simulink model "ActuatorRatingModel"  (R2024a)
settings: Solver=VariableStepAuto  StartTime=0.0  StopTime=simT  MaxStep=1e-3  MinStep=1e-4  RelTol=1e-3
PostLoadFcn:
  | run('ParametricRobotParameters')
  | run('ParametricGripperPayloadsParameters.m');
  | simT = 2;
  | load('configModelWorkspace.mat');
  | jointDataBus = jointDataBusCreator;
undefined symbols (not defined in the file): ParametricRobot, positionLimits, timeScale, velocityLimits, waypoints, X, Y, Z
libraries: nesl_utility x7, simulink x6, sm_lib x4
settings Model: Creator=jjha  LastModifiedBy=abirdas
settings OptimizationCC: ReuseModelBlockBuffer=off
settings RTWCC: GPUComputeCapability=3.5
settings SimscapeCC: SimscapeLogType=all

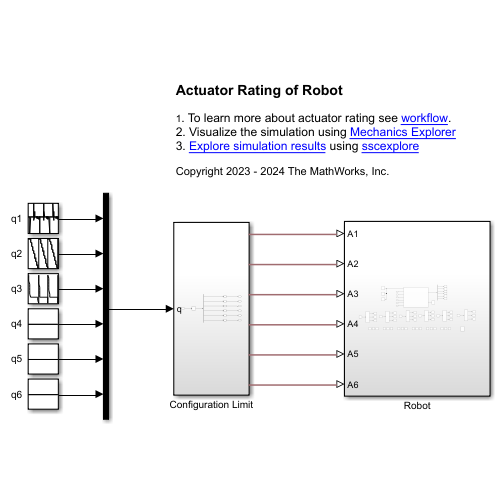
[thumbnail: Simulink's stored preview of the top-level diagram]
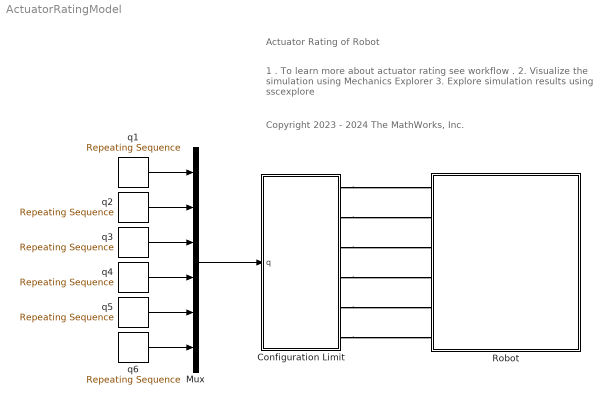
== system ActuatorRatingModel ==
  note: Copyright 2023 - 2024 The MathWorks, Inc.
  note: Actuator Rating of Robot
  note: 1 . To learn more about actuator rating see workflow .
      | 2. Visualize the simulation using Mechanics Explorer
      | 3. Explore simulation results using sscexplore
  Configuration Limit : Subsystem
  Mux : Mux  Inputs=6
  Robot : Subsystem
  q1 : simulink/Sources/Repeating Sequence  rep_seq_t=[1 : length(waypoints)] * timeScale  rep_seq_y=waypoints(1,:)
  q2 : simulink/Sources/Repeating Sequence  rep_seq_t=[1 : length(waypoints)] * timeScale  rep_seq_y=waypoints(2,:)
  q3 : simulink/Sources/Repeating Sequence  rep_seq_t=[1 : length(waypoints)] * timeScale  rep_seq_y=waypoints(3,:)
  q4 : simulink/Sources/Repeating Sequence  rep_seq_t=[1 : length(waypoints)] * timeScale  rep_seq_y=waypoints(4,:)
  q5 : simulink/Sources/Repeating Sequence  rep_seq_t=[1 : length(waypoints)] * timeScale  rep_seq_y=waypoints(5,:)
  q6 : simulink/Sources/Repeating Sequence  rep_seq_t=[1 : length(waypoints)] * timeScale  rep_seq_y=waypoints(6,:)
  wires:
  q1/1 -> Mux/1
  Mux/1 -> Configuration Limit/1(q)
  q6/1 -> Mux/6
  q3/1 -> Mux/3
  q5/1 -> Mux/5
  q2/1 -> Mux/2
  q4/1 -> Mux/4
  connections:
  Configuration Limit/RConn5 -- Robot/LConn5
  Configuration Limit/RConn6 -- Robot/LConn6
  Configuration Limit/RConn4 -- Robot/LConn4
  Configuration Limit/RConn1 -- Robot/LConn1
  Configuration Limit/RConn3 -- Robot/LConn3
  Configuration Limit/RConn2 -- Robot/LConn2

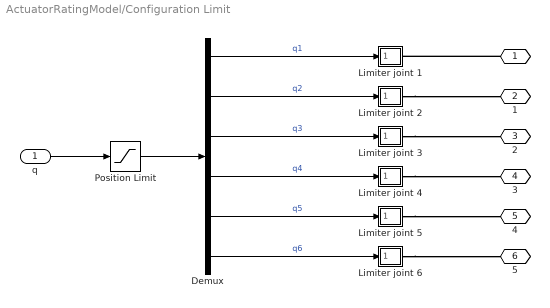
== system ActuatorRatingModel/Configuration Limit ==
  q : Inport
  Demux : Demux  Outputs=6
  Limiter joint 1 : Subsystem  mask(Limiter){maxVel=velocityLimits(1), maxAcc=0.1}
      mask prompts: maxVel "Max velocity of joint (rad/s)"; maxAcc "max acceleration of joint (rad/s^2)"
      mask help: Limit the velocity and acceleration of joints.
      mask DialogControl ParameterGroupVar Prompt: Limits
  Limiter joint 2 : Subsystem  mask(Limiter){maxVel=velocityLimits(2), maxAcc=0.1}
      mask prompts: maxVel "Max velocity of joint (rad/s)"; maxAcc "max acceleration of joint (rad/s^2)"
      mask help: Limit the velocity and acceleration of joints.
      mask DialogControl ParameterGroupVar Prompt: Limits
  Limiter joint 3 : Subsystem  mask(Limiter){maxVel=velocityLimits(3), maxAcc=0.1}
      mask prompts: maxVel "Max velocity of joint (rad/s)"; maxAcc "max acceleration of joint (rad/s^2)"
      mask help: Limit the velocity and acceleration of joints.
      mask DialogControl ParameterGroupVar Prompt: Limits
  Limiter joint 4 : Subsystem  mask(Limiter){maxVel=velocityLimits(4), maxAcc=0.1}
      mask prompts: maxVel "Max velocity of joint (rad/s)"; maxAcc "max acceleration of joint (rad/s^2)"
      mask help: Limit the velocity and acceleration of joints.
      mask DialogControl ParameterGroupVar Prompt: Limits
  Limiter joint 5 : Subsystem  mask(Limiter){maxVel=velocityLimits(5), maxAcc=0.1}
      mask prompts: maxVel "Max velocity of joint (rad/s)"; maxAcc "max acceleration of joint (rad/s^2)"
      mask help: Limit the velocity and acceleration of joints.
      mask DialogControl ParameterGroupVar Prompt: Limits
  Limiter joint 6 : Subsystem  mask(Limiter){maxVel=velocityLimits(6), maxAcc=0.1}
      mask prompts: maxVel "Max velocity of joint (rad/s)"; maxAcc "max acceleration of joint (rad/s^2)"
      mask help: Limit the velocity and acceleration of joints.
      mask DialogControl ParameterGroupVar Prompt: Limits
  Position Limit : Saturate  UpperLimit=positionLimits(:, 2)  LowerLimit=positionLimits(:, 1)
  " " : PMIOPort  Side=Right
  " 1" : PMIOPort  Port=2  Side=Right
  " 2" : PMIOPort  Port=3  Side=Right
  " 3" : PMIOPort  Port=4  Side=Right
  " 4" : PMIOPort  Port=5  Side=Right
  " 5" : PMIOPort  Port=6  Side=Right
  wires:
  Demux/1 -> Limiter joint 1/1(" ")  "q1"
  q/1 -> Position Limit/1
  Demux/2 -> Limiter joint 2/1(" ")  "q2"
  Demux/3 -> Limiter joint 3/1(" ")  "q3"
  Demux/4 -> Limiter joint 4/1(" ")  "q4"
  Demux/5 -> Limiter joint 5/1(" ")  "q5"
  Demux/6 -> Limiter joint 6/1(" ")  "q6"
  Position Limit/1 -> Demux/1
  connections:
  " "/RConn1 -- Limiter joint 1/RConn1
  Limiter joint 2/RConn1 -- " 1"/RConn1
  Limiter joint 3/RConn1 -- " 2"/RConn1
  Limiter joint 4/RConn1 -- " 3"/RConn1
  Limiter joint 5/RConn1 -- " 4"/RConn1
  Limiter joint 6/RConn1 -- " 5"/RConn1

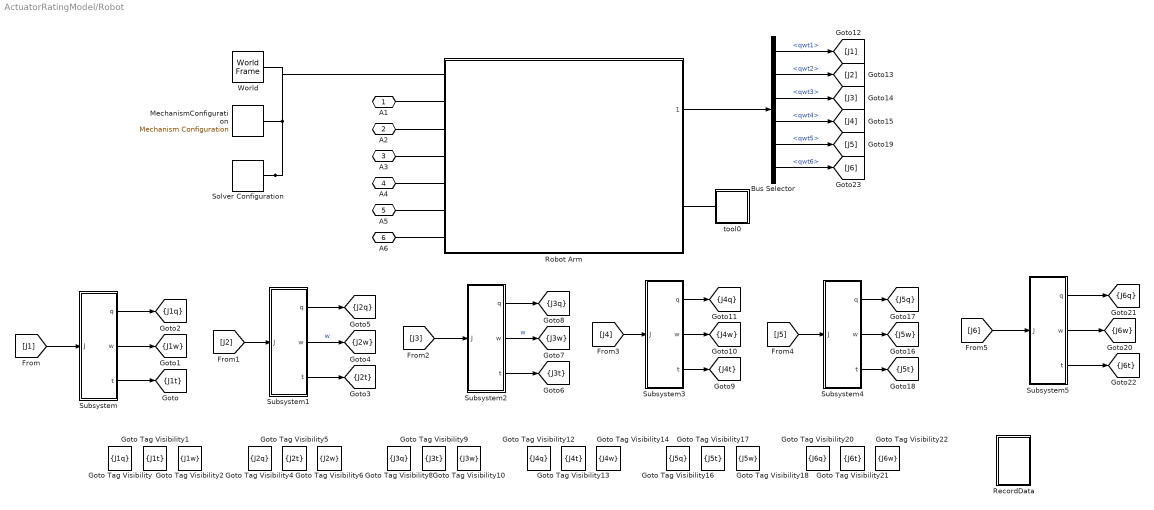
== system ActuatorRatingModel/Robot ==
  Bus Selector : BusSelector  OutputSignals=qwt1,qwt2,qwt3,qwt4,qwt5,qwt6
  Goto Tag Visibility : GotoTagVisibility  GotoTag=J1q
  Goto Tag Visibility1 : GotoTagVisibility  GotoTag=J1t
  Goto Tag Visibility10 : GotoTagVisibility  GotoTag=J3w
  Goto Tag Visibility12 : GotoTagVisibility  GotoTag=J4q
  Goto Tag Visibility13 : GotoTagVisibility  GotoTag=J4t
  Goto Tag Visibility14 : GotoTagVisibility  GotoTag=J4w
  Goto Tag Visibility16 : GotoTagVisibility  GotoTag=J5q
  Goto Tag Visibility17 : GotoTagVisibility  GotoTag=J5t
  Goto Tag Visibility18 : GotoTagVisibility  GotoTag=J5w
  Goto Tag Visibility2 : GotoTagVisibility  GotoTag=J1w
  Goto Tag Visibility20 : GotoTagVisibility  GotoTag=J6q
  Goto Tag Visibility21 : GotoTagVisibility  GotoTag=J6t
  Goto Tag Visibility22 : GotoTagVisibility  GotoTag=J6w
  Goto Tag Visibility4 : GotoTagVisibility  GotoTag=J2q
  Goto Tag Visibility5 : GotoTagVisibility  GotoTag=J2t
  Goto Tag Visibility6 : GotoTagVisibility  GotoTag=J2w
  Goto Tag Visibility8 : GotoTagVisibility  GotoTag=J3q
  Goto Tag Visibility9 : GotoTagVisibility  GotoTag=J3t
  MechanismConfiguration : sm_lib/Utilities/Mechanism Configuration  UniformGravity=Constant  GravityVector=[0 0 -9.80665]  GravityVectorUnits=m/s^2  LinearizationDelta=0.001  JointModeTransitionNonlinearIterations=2
  RecordData : Subsystem
  Robot Arm : Subsystem  ReferencedSubsystem=ParametricRobotSubsystem  workflow=ones(1,6)*2
  Solver Configuration : nesl_utility/Solver Configuration  PhysicalDomain=network_engine_domain  SubClassName=solver  LeftPortType=input  RightPortType=generic  Tones=[]  Harmonics=[]  SimulateNoise=off  Profile=off  UseLocalSampling=off  EnableSwitchedLinearOptims=on  FrequencyDomain=off  UseCCode=off  RelTol=0.001  AbsTol=0.001  MinStep=1e-09  ToWorkspace=off  RevertToSquareIcSolve=off  NumHomotopyIterations=100  PhasorMode=off  PhasorModeNumHarmonics=1  ConsistencySolver=NEWTON_XTOL_AFTER_FTOL  IndexReductionMethod=DerivativeReplacement  DoDC=off  ResidualTolerance=1e-09  ConsistencyTolSource=GLOBAL  ConsistencyAbsTol=0.001  ConsistencyRelTol=0.001  ConsistencyTolFactor=0.001  UseLocalSolver=off  LocalSolverChoice=NE_BACKWARD_EULER_ADVANCER  ResolveIndetEquations=on  FunctionEvalNumThread=1  LocalSolverSampleTime=0.001  DoFixedCost=off  MaxNonlinIter=3  MaxModeIter=2  ComputeImpulses=off  ImpulseIterations=2  LinearAlgebra=auto  LinearAlgebraNumThread=0  EquationFormulation=NE_TIME_EF  DelaysMemoryBudget=1024  AutomaticFiltering=on  FilteringTimeConstant=0.001  PartitionStorageMethod=AS_NEEDED  PartitionMemoryBudget=1024  PartitionMethod=ROBUST  MultibodyUseLocalSolver=off  MultibodyLocalSolverChoice=ODE1  MultibodyLocalSolverSampleTime=0.001
  Subsystem : Subsystem
  Subsystem1 : Subsystem
  Subsystem2 : Subsystem
  Subsystem3 : Subsystem
  Subsystem4 : Subsystem
  Subsystem5 : Subsystem
  World : sm_lib/Frames and Transforms/World Frame
  tool0 : Subsystem
  A1 : PMIOPort  Side=Left
  A2 : PMIOPort  Port=2  Side=Left
  A3 : PMIOPort  Port=3  Side=Left
  A4 : PMIOPort  Port=4  Side=Left
  A5 : PMIOPort  Port=5  Side=Left
  A6 : PMIOPort  Port=6  Side=Left
  tag scope: J1q=scoped, J1t=scoped, J1w=scoped, J2q=scoped, J2t=scoped, J2w=scoped, J3q=scoped, J3t=scoped, J3w=scoped, J4q=scoped, J4t=scoped, J4w=scoped, J5q=scoped, J5t=scoped, J5w=scoped, J6q=scoped, J6t=scoped, J6w=scoped
  wires:
  Subsystem4/1(q) -> [J5q]
  Subsystem/2(w) -> [J1w]
  Subsystem5/2(w) -> [J6w]
  [J4] -> Subsystem3/1(J)
  Subsystem5/3(t) -> [J6t]
  Subsystem/3(t) -> [J1t]
  Subsystem4/2(w) -> [J5w]
  [J6] -> Subsystem5/1(J)
  [J3] -> Subsystem2/1(J)
  Subsystem5/1(q) -> [J6q]
  Subsystem1/1(q) -> [J2q]
  [J1] -> Subsystem/1(J)
  [J2] -> Subsystem1/1(J)
  Subsystem/1(q) -> [J1q]
  Subsystem3/1(q) -> [J4q]
  Subsystem3/2(w) -> [J4w]
  Subsystem4/3(t) -> [J5t]
  Subsystem2/1(q) -> [J3q]
  Subsystem2/2(w) -> [J3w]  "w"
  [J5] -> Subsystem4/1(J)
  Subsystem2/3(t) -> [J3t]
  Subsystem1/2(w) -> [J2w]  "w"
  Subsystem1/3(t) -> [J2t]
  Subsystem3/3(t) -> [J4t]
  Bus Selector/1 -> [J1]  "<qwt1>"
  Bus Selector/2 -> [J2]  "<qwt2>"
  Bus Selector/3 -> [J3]  "<qwt3>"
  Bus Selector/4 -> [J4]  "<qwt4>"
  Bus Selector/5 -> [J5]  "<qwt5>"
  Bus Selector/6 -> [J6]  "<qwt6>"
  Robot Arm/1 -> Bus Selector/1
  connections:
  Solver Configuration/RConn1 -- Robot Arm/LConn1 -- World/RConn1 -- MechanismConfiguration/RConn1
  A5/RConn1 -- Robot Arm/LConn6
  tool0/LConn1 -- Robot Arm/RConn1
  A4/RConn1 -- Robot Arm/LConn5
  A3/RConn1 -- Robot Arm/LConn4
  A1/RConn1 -- Robot Arm/LConn2
  A2/RConn1 -- Robot Arm/LConn3
  A6/RConn1 -- Robot Arm/LConn7

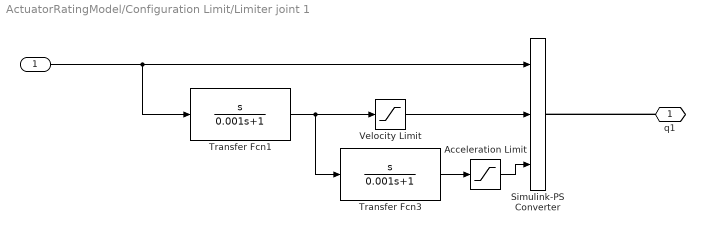
== system ActuatorRatingModel/Configuration Limit/Limiter joint 1 ==
  " " : Inport
  Acceleration Limit : Saturate  UpperLimit=maxAcc  LowerLimit=-maxAcc
  Simulink-PS Converter : nesl_utility/Simulink-PS Converter  PhysicalDomain=network_engine_domain  SubClassName=ps_input  LeftPortType=input  RightPortType=output  PseudoPeriodic=off  Frequencies=[]  NoiseDistribution=none  NoiseParameters=[]  Unit=rad  AffineConversion=off  FilteringAndDerivatives=provide  SimscapeFilterOrder=1  InputFilterTimeConstant=0.001  UdotUserProvided=2
  Transfer Fcn1 : TransferFcn  Numerator=[1 0]  Denominator=[0.001 1]
  Transfer Fcn3 : TransferFcn  Numerator=[1 0]  Denominator=[0.001 1]
  Velocity Limit : Saturate  UpperLimit=maxVel  LowerLimit=-maxVel
  q1 : PMIOPort  Side=Right
  wires:
  " "/1 -> Transfer Fcn1/1, Simulink-PS Converter/1
  Transfer Fcn1/1 -> Transfer Fcn3/1, Velocity Limit/1
  Velocity Limit/1 -> Simulink-PS Converter/2
  Transfer Fcn3/1 -> Acceleration Limit/1
  Acceleration Limit/1 -> Simulink-PS Converter/3
  connections:
  q1/RConn1 -- Simulink-PS Converter/RConn1

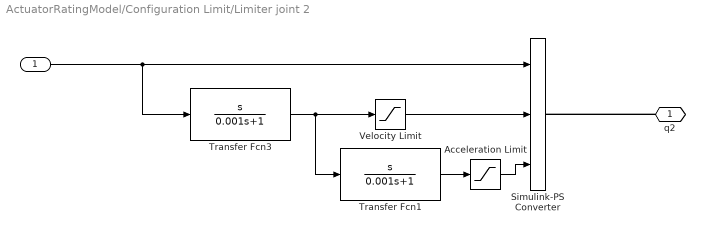
== system ActuatorRatingModel/Configuration Limit/Limiter joint 2 ==
  " " : Inport
  Acceleration Limit : Saturate  UpperLimit=maxAcc  LowerLimit=-maxAcc
  Simulink-PS Converter : nesl_utility/Simulink-PS Converter  PhysicalDomain=network_engine_domain  SubClassName=ps_input  LeftPortType=input  RightPortType=output  PseudoPeriodic=off  Frequencies=[]  NoiseDistribution=none  NoiseParameters=[]  Unit=rad  AffineConversion=off  FilteringAndDerivatives=provide  SimscapeFilterOrder=1  InputFilterTimeConstant=0.001  UdotUserProvided=2
  Transfer Fcn1 : TransferFcn  Numerator=[1 0]  Denominator=[0.001 1]
  Transfer Fcn3 : TransferFcn  Numerator=[1 0]  Denominator=[0.001 1]
  Velocity Limit : Saturate  UpperLimit=maxVel  LowerLimit=-maxVel
  q2 : PMIOPort  Side=Right
  wires:
  Transfer Fcn1/1 -> Acceleration Limit/1
  Transfer Fcn3/1 -> Transfer Fcn1/1, Velocity Limit/1
  " "/1 -> Transfer Fcn3/1, Simulink-PS Converter/1
  Velocity Limit/1 -> Simulink-PS Converter/2
  Acceleration Limit/1 -> Simulink-PS Converter/3
  connections:
  q2/RConn1 -- Simulink-PS Converter/RConn1

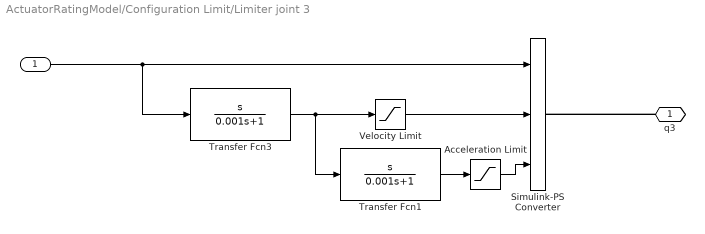
== system ActuatorRatingModel/Configuration Limit/Limiter joint 3 ==
  " " : Inport
  Acceleration Limit : Saturate  UpperLimit=maxAcc  LowerLimit=-maxAcc
  Simulink-PS Converter : nesl_utility/Simulink-PS Converter  PhysicalDomain=network_engine_domain  SubClassName=ps_input  LeftPortType=input  RightPortType=output  PseudoPeriodic=off  Frequencies=[]  NoiseDistribution=none  NoiseParameters=[]  Unit=rad  AffineConversion=off  FilteringAndDerivatives=provide  SimscapeFilterOrder=1  InputFilterTimeConstant=0.001  UdotUserProvided=2
  Transfer Fcn1 : TransferFcn  Numerator=[1 0]  Denominator=[0.001 1]
  Transfer Fcn3 : TransferFcn  Numerator=[1 0]  Denominator=[0.001 1]
  Velocity Limit : Saturate  UpperLimit=maxVel  LowerLimit=-maxVel
  q3 : PMIOPort  Side=Right
  wires:
  " "/1 -> Transfer Fcn3/1, Simulink-PS Converter/1
  Transfer Fcn3/1 -> Transfer Fcn1/1, Velocity Limit/1
  Velocity Limit/1 -> Simulink-PS Converter/2
  Transfer Fcn1/1 -> Acceleration Limit/1
  Acceleration Limit/1 -> Simulink-PS Converter/3
  connections:
  q3/RConn1 -- Simulink-PS Converter/RConn1

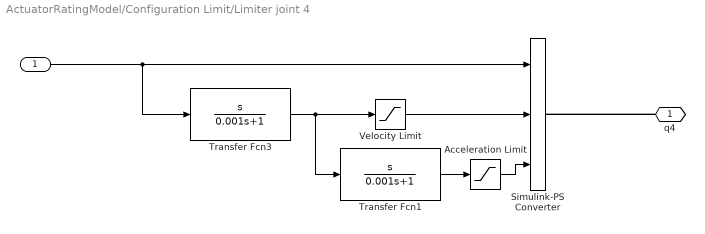
== system ActuatorRatingModel/Configuration Limit/Limiter joint 4 ==
  " " : Inport
  Acceleration Limit : Saturate  UpperLimit=maxAcc  LowerLimit=-maxAcc
  Simulink-PS Converter : nesl_utility/Simulink-PS Converter  PhysicalDomain=network_engine_domain  SubClassName=ps_input  LeftPortType=input  RightPortType=output  PseudoPeriodic=off  Frequencies=[]  NoiseDistribution=none  NoiseParameters=[]  Unit=rad  AffineConversion=off  FilteringAndDerivatives=provide  SimscapeFilterOrder=1  InputFilterTimeConstant=0.001  UdotUserProvided=2
  Transfer Fcn1 : TransferFcn  Numerator=[1 0]  Denominator=[0.001 1]
  Transfer Fcn3 : TransferFcn  Numerator=[1 0]  Denominator=[0.001 1]
  Velocity Limit : Saturate  UpperLimit=maxVel  LowerLimit=-maxVel
  q4 : PMIOPort  Side=Right
  wires:
  Acceleration Limit/1 -> Simulink-PS Converter/3
  Transfer Fcn1/1 -> Acceleration Limit/1
  Velocity Limit/1 -> Simulink-PS Converter/2
  Transfer Fcn3/1 -> Transfer Fcn1/1, Velocity Limit/1
  " "/1 -> Transfer Fcn3/1, Simulink-PS Converter/1
  connections:
  q4/RConn1 -- Simulink-PS Converter/RConn1

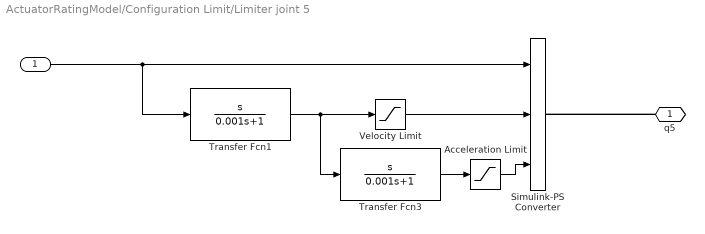
== system ActuatorRatingModel/Configuration Limit/Limiter joint 5 ==
  " " : Inport
  Acceleration Limit : Saturate  UpperLimit=maxAcc  LowerLimit=-maxAcc
  Simulink-PS Converter : nesl_utility/Simulink-PS Converter  PhysicalDomain=network_engine_domain  SubClassName=ps_input  LeftPortType=input  RightPortType=output  PseudoPeriodic=off  Frequencies=[]  NoiseDistribution=none  NoiseParameters=[]  Unit=rad  AffineConversion=off  FilteringAndDerivatives=provide  SimscapeFilterOrder=1  InputFilterTimeConstant=0.001  UdotUserProvided=2
  Transfer Fcn1 : TransferFcn  Numerator=[1 0]  Denominator=[0.001 1]
  Transfer Fcn3 : TransferFcn  Numerator=[1 0]  Denominator=[0.001 1]
  Velocity Limit : Saturate  UpperLimit=maxVel  LowerLimit=-maxVel
  q5 : PMIOPort  Side=Right
  wires:
  " "/1 -> Transfer Fcn1/1, Simulink-PS Converter/1
  Transfer Fcn1/1 -> Transfer Fcn3/1, Velocity Limit/1
  Velocity Limit/1 -> Simulink-PS Converter/2
  Transfer Fcn3/1 -> Acceleration Limit/1
  Acceleration Limit/1 -> Simulink-PS Converter/3
  connections:
  q5/RConn1 -- Simulink-PS Converter/RConn1

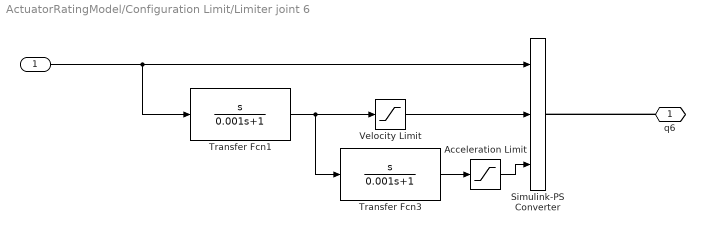
== system ActuatorRatingModel/Configuration Limit/Limiter joint 6 ==
  " " : Inport
  Acceleration Limit : Saturate  UpperLimit=maxAcc  LowerLimit=-maxAcc
  Simulink-PS Converter : nesl_utility/Simulink-PS Converter  PhysicalDomain=network_engine_domain  SubClassName=ps_input  LeftPortType=input  RightPortType=output  PseudoPeriodic=off  Frequencies=[]  NoiseDistribution=none  NoiseParameters=[]  Unit=rad  AffineConversion=off  FilteringAndDerivatives=provide  SimscapeFilterOrder=1  InputFilterTimeConstant=0.001  UdotUserProvided=2
  Transfer Fcn1 : TransferFcn  Numerator=[1 0]  Denominator=[0.001 1]
  Transfer Fcn3 : TransferFcn  Numerator=[1 0]  Denominator=[0.001 1]
  Velocity Limit : Saturate  UpperLimit=maxVel  LowerLimit=-maxVel
  q6 : PMIOPort  Side=Right
  wires:
  Acceleration Limit/1 -> Simulink-PS Converter/3
  Transfer Fcn3/1 -> Acceleration Limit/1
  Velocity Limit/1 -> Simulink-PS Converter/2
  Transfer Fcn1/1 -> Transfer Fcn3/1, Velocity Limit/1
  " "/1 -> Transfer Fcn1/1, Simulink-PS Converter/1
  connections:
  q6/RConn1 -- Simulink-PS Converter/RConn1

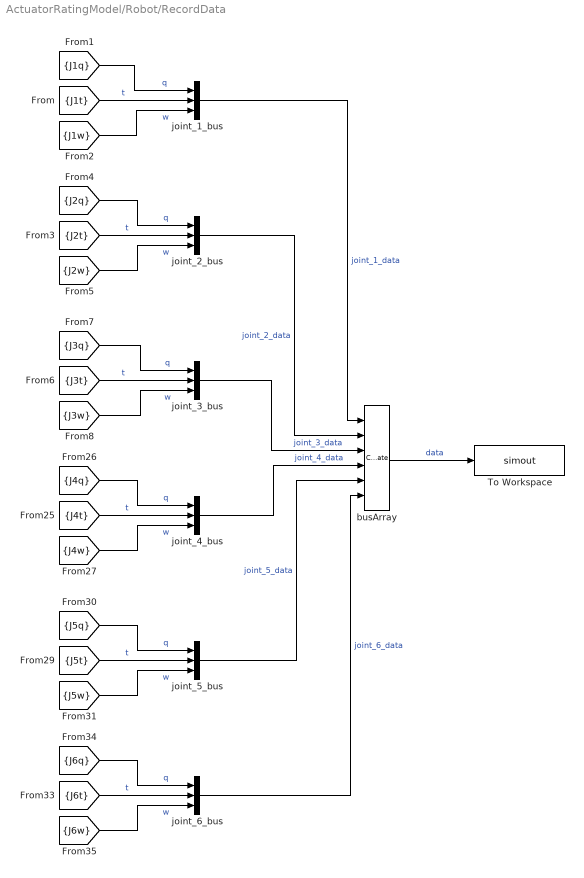
== system ActuatorRatingModel/Robot/RecordData ==
  To Workspace : ToWorkspace  VariableName=simout  SaveFormat=Timeseries  SampleTime=-1
  busArray : Concatenate  NumInputs=6  Mode=Multidimensional array
  joint_1_bus : BusCreator  Inputs=3  OutDataTypeStr=Bus: jointDataBus  NonVirtualBus=on
  joint_2_bus : BusCreator  Inputs=3  OutDataTypeStr=Bus: jointDataBus  NonVirtualBus=on
  joint_3_bus : BusCreator  Inputs=3  OutDataTypeStr=Bus: jointDataBus  NonVirtualBus=on
  joint_4_bus : BusCreator  Inputs=3  OutDataTypeStr=Bus: jointDataBus  NonVirtualBus=on
  joint_5_bus : BusCreator  Inputs=3  OutDataTypeStr=Bus: jointDataBus  NonVirtualBus=on
  joint_6_bus : BusCreator  Inputs=3  OutDataTypeStr=Bus: jointDataBus  NonVirtualBus=on
  wires:
  [J5q] -> joint_5_bus/1  "q"
  [J6q] -> joint_6_bus/1  "q"
  [J4w] -> joint_4_bus/3  "w"
  joint_2_bus/1 -> busArray/2  "joint_2_data"
  [J3w] -> joint_3_bus/3  "w"
  [J5w] -> joint_5_bus/3  "w"
  [J5t] -> joint_5_bus/2  "t"
  joint_1_bus/1 -> busArray/1  "joint_1_data"
  joint_5_bus/1 -> busArray/5  "joint_5_data"
  [J1w] -> joint_1_bus/3  "w"
  [J3t] -> joint_3_bus/2  "t"
  [J3q] -> joint_3_bus/1  "q"
  [J4t] -> joint_4_bus/2  "t"
  joint_6_bus/1 -> busArray/6  "joint_6_data"
  [J1t] -> joint_1_bus/2  "t"
  [J1q] -> joint_1_bus/1  "q"
  joint_4_bus/1 -> busArray/4  "joint_4_data"
  joint_3_bus/1 -> busArray/3  "joint_3_data"
  [J6w] -> joint_6_bus/3  "w"
  busArray/1 -> To Workspace/1  "data"
  [J2q] -> joint_2_bus/1  "q"
  [J6t] -> joint_6_bus/2  "t"
  [J2w] -> joint_2_bus/3  "w"
  [J2t] -> joint_2_bus/2  "t"
  [J4q] -> joint_4_bus/1  "q"

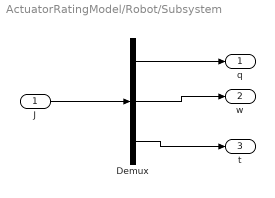
== system ActuatorRatingModel/Robot/Subsystem ==
  J : Inport
  Demux : Demux  Outputs=3
  q : Outport
  w : Outport  Port=2
  t : Outport  Port=3
  wires:
  Demux/1 -> q/1
  Demux/2 -> w/1
  J/1 -> Demux/1
  Demux/3 -> t/1

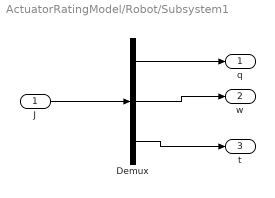
== system ActuatorRatingModel/Robot/Subsystem1 ==
  J : Inport
  Demux : Demux  Outputs=3
  q : Outport
  w : Outport  Port=2
  t : Outport  Port=3
  wires:
  Demux/3 -> t/1
  J/1 -> Demux/1
  Demux/2 -> w/1
  Demux/1 -> q/1

== system ActuatorRatingModel/Robot/Subsystem2 ==
  J : Inport
  Demux : Demux  Outputs=3
  q : Outport
  w : Outport  Port=2
  t : Outport  Port=3
  wires:
  Demux/1 -> q/1
  Demux/2 -> w/1
  J/1 -> Demux/1
  Demux/3 -> t/1

== system ActuatorRatingModel/Robot/Subsystem3 ==
  J : Inport
  Demux : Demux  Outputs=3
  q : Outport
  w : Outport  Port=2
  t : Outport  Port=3
  wires:
  Demux/3 -> t/1
  J/1 -> Demux/1
  Demux/2 -> w/1
  Demux/1 -> q/1

== system ActuatorRatingModel/Robot/Subsystem4 ==
  J : Inport
  Demux : Demux  Outputs=3
  q : Outport
  w : Outport  Port=2
  t : Outport  Port=3
  wires:
  Demux/1 -> q/1
  Demux/2 -> w/1
  J/1 -> Demux/1
  Demux/3 -> t/1

== system ActuatorRatingModel/Robot/Subsystem5 ==
  J : Inport
  Demux : Demux  Outputs=3
  q : Outport
  w : Outport  Port=2
  t : Outport  Port=3
  wires:
  Demux/3 -> t/1
  J/1 -> Demux/1
  Demux/2 -> w/1
  Demux/1 -> q/1

== system ActuatorRatingModel/Robot/tool0 ==
  Payload Mass : sm_lib/Body Elements/Brick Solid  BrickDimensions=[ParametricRobot.Payloads.Length ParametricRobot.Payloads.Width ParametricRobot.Payloads.Thickness]  BrickDimensionsUnits=m  ExportEntireGeometry=off  InertiaType=CalculateFromGeometry  BasedOnType=Density  Density=ParametricRobot.Payloads.Density  DensityUnits=kg/m^3  Mass=1  MassUnits=kg  CenterOfMass=[0 0 0]  CenterOfMassUnits=m  MomentsOfInertia=[1 1 1]  MomentsOfInertiaUnits=kg*m^2  ProductsOfInertia=[0 0 0]  ProductsOfInertiaUnits=kg*m^2  GraphicType=FromGeometry  MarkerShape=Sphere  MarkerSize=10  GraphicVisPropType=SimpleVisualProperties  GraphicDiffuseColor=[0.8 0.2 0.1]  GraphicOpacity=1.0  GraphicSpecularColor=[0.5 0.5 0.5 1.0]  GraphicAmbientColor=[0.15 0.15 0.15 1.0]  GraphicEmissiveColor=[0.0 0.0 0.0 1.0]  GraphicShininess=75  DoExposeReferenceFrame=off  SerializedFrames=<Frames><Frame><Id>Frame1</Id><Value><Name>F1</Name><Origin><Source>GeometricFeature</Source><FeatureName>-y surface</FeatureName></Origin><PrimaryAxis><DefinedDirection>+Z</DefinedDirection><Source>ReferenceFrame</Source><SourceDirection>+Z</SourceDirection><FeatureName></FeatureName></PrimaryAxis><SecondaryAxis><DefinedDirection>+X</DefinedDirection><Source>ReferenceFrame</Source><SourceDirection>+X</SourceDirection><FeatureName></FeatureName></SecondaryAxis></Value></Frame></Frames>
  Rigid Transform : sm_lib/Frames and Transforms/Rigid Transform  RotationMethod=StandardAxis  FollAlignAxisA=+X  BaseAlignAxisA=+Y  FollAlignAxisB=+Y  BaseAlignAxisB=+Z  RotationStandardAxis=+X  RotationAngle=90  RotationAngleUnits=deg  RotationArbitraryAxis=[0 0 1]  RotationSequenceAxes=FollowerAxes  RotationSequence=XYX  RotationSequenceAngles=[0 0 0]  RotationSequenceAnglesUnits=deg  RotationMatrix=[1 0 0; 0 1 0; 0 0 1]  Quaternion=[1 0 0 0]  TranslationMethod=None  TranslationCartesianOffset=[0 0 0]  TranslationCartesianOffsetUnits=m  TranslationStandardAxis=-Z  TranslationStandardOffset=15  TranslationStandardOffsetUnits=mm  TranslationROffset=0  TranslationROffsetUnits=m  TranslationThetaOffset=0  TranslationThetaOffsetUnits=deg  TranslationZOffset=0  TranslationZOffsetUnits=m
  F : PMIOPort  Side=Left
  connections:
  Rigid Transform/LConn1 -- F/RConn1
  Payload Mass/LConn1 -- Rigid Transform/RConn1
